simulink model "IEEE14Bus"  (R2024a)
settings: Solver=VariableStepAuto  StartTime=0.0  StopTime=10.0  RelTol=1e-3
values from neighbouring files (symbols this model uses):
  D1 = 2    [IEEE14Bus_params.m]
  M = 2*5.06    (= 10.12)    [IEEE14bus.m]    (also in IEEE14bus_revision.m; IEEE14bus_revision_new.m; IEEE14bus_revision_old.m; IEEE68withLocalSys14.m)
  Xd = 1.25    [IEEE14bus.m]    (also in IEEE14bus_revision.m; IEEE14bus_revision_new.m; IEEE14bus_revision_old.m; IEEE68withLocalSys14.m)
  Xq = 1.22    [IEEE14bus.m]    (also in IEEE14bus_revision.m; IEEE14bus_revision_new.m; IEEE14bus_revision_old.m; IEEE68withLocalSys14.m)
undefined symbols (not defined in the file or in its folder): ddTdo, ddTqo, ddXd, ddXq, Delta, dTdo, dXd, F, T1, T2, T3, T4, T5, T6, Xl
libraries: spsGroundLib x3, spsThreePhaseSeriesRLCBranchLib x3, spsThreePhaseParallelRLCLoadLib x2, spsLoadFlowBusLib x2, spsThreePhaseVIMeasurementLib x2, spsThreePhaseSourceLib x1, spsThreePhaseFaultLib x1, spsDC1AExcitationSystemLib x1, spsGenericPowerSystemStabilizerLib x1, spsST1AExcitationSystemLib x1, spsSynchronousMachinepuStandardLib x1, spsThreePhaseTransformerTwoWindingsLib x1
settings Model: Creator=byeonghwalee  LastModifiedBy=byeonghwalee

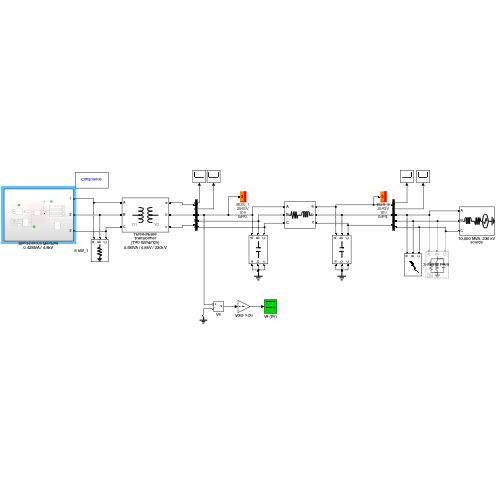
[thumbnail: Simulink's stored preview of the top-level diagram]
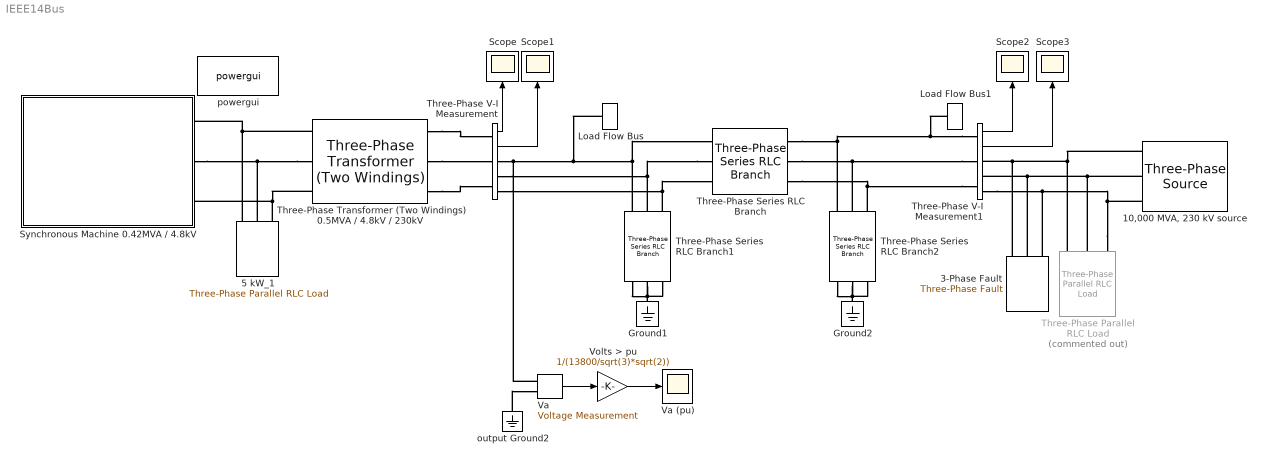
== system IEEE14Bus ==
  "10,000 MVA, 230 kV source" : spsThreePhaseSourceLib/Three-Phase Source  InternalConnection=Yg  VoltagePhases=off  Voltage=(230000)*1.00006  PhaseAngle=-0.77547  Voltage_phases=[25e3 25e3 25e3]/sqrt(3)  PhaseAngles_phases=[0 -120 +120]  Frequency=60  NonIdealSource=on  SpecifyImpedance=on  Resistance=0.529  Inductance=0.0140  ShortCircuitLevel=10000e6  BaseVoltage=230e3  XRratio=10  BusType=swing  Pref=0  Qref=0  Prefabc=[10e3, 10e3, 10e3]  Qrefabc=[0, 0, 0]  Qmin=-Inf  Qmax=Inf
  3-Phase Fault : spsThreePhaseFaultLib/Three-Phase Fault  InitialStates=0  FaultA=on  FaultB=on  FaultC=on  GroundFault=on  SwitchTimes=[3]  External=off  SwitchStatus=NaN  FaultResistance=1e-3  GroundResistance=1e-3  SnubberResistance=inf  SnubberCapacitance=inf  Measurements=None
  5 kW_1 : spsThreePhaseParallelRLCLoadLib/Three-Phase Parallel RLC Load  LConnTagsString=A|B|C  Configuration=Y (grounded)  NominalVoltage=230e3  Vabc=[1e3 1e3 1e3]  Vabcp=[1e3 1e3 1e3]  NominalFrequency=60  UnbalancedPower=off  ActivePower=100e3  InductivePower=0  CapacitivePower=0  Pabc=[10e3 9e3 11e3]  QLabc=[100 90 110]  QCabc=[100 90 110]  Pabcp=[10e3 9e3 11e3]  QLabcp=[100 90 110]  QCabcp=[100 90 110]  Measurements=None  LoadType=constant Z
  Ground1 : spsGroundLib/Ground  LConnTagsString=a
  Ground2 : spsGroundLib/Ground  LConnTagsString=a
  Load Flow Bus : spsLoadFlowBusLib/Load Flow Bus  LConnTagsString=a  Phases=single  Connectors=on one side  ID=BUS_1  Vbase=25e3  Vref=1  Vangle=0  VLF=1  VLFb=1  VLFc=1  angleLF=0  angleLFb=0  angleLFc=0
  Load Flow Bus1 : spsLoadFlowBusLib/Load Flow Bus  LConnTagsString=a  Phases=single  Connectors=on one side  ID=BUS_2  Vbase=25e3  Vref=1  Vangle=0  VLF=1  VLFb=1  VLFc=1  angleLF=0  angleLFb=0  angleLFc=0
  Scope{,1..3} (4 alike) : Scope
  Synchronous Machine 0.42MVA / 4.8kV : Subsystem
  Three-Phase Parallel RLC Load : spsThreePhaseParallelRLCLoadLib/Three-Phase Parallel RLC Load  Commented=on  LConnTagsString=A|B|C  Configuration=Y (grounded)  NominalVoltage=1000  Vabc=[1e3 1e3 1e3]  Vabcp=[1e3 1e3 1e3]  NominalFrequency=60  UnbalancedPower=off  ActivePower=10e3  InductivePower=100  CapacitivePower=100  Pabc=[10e3 9e3 11e3]  QLabc=[100 90 110]  QCabc=[100 90 110]  Pabcp=[10e3 9e3 11e3]  QLabcp=[100 90 110]  QCabcp=[100 90 110]  Measurements=None  LoadType=constant Z
  Three-Phase Series RLC Branch : spsThreePhaseSeriesRLCBranchLib/Three-Phase Series RLC Branch  LConnTagsString=A|B|C  RConnTagsString=A|B|C  BranchType=RL  Resistance=0.1375  Inductance=0.0698  Capacitance=1e-6  Measurements=None
  Three-Phase Series RLC Branch1 : spsThreePhaseSeriesRLCBranchLib/Three-Phase Series RLC Branch  LConnTagsString=A|B|C  RConnTagsString=A|B|C  BranchType=C  Resistance=1  Inductance=1e-3  Capacitance=(7.9377e-6)/2  Measurements=None
  Three-Phase Series RLC Branch2 : spsThreePhaseSeriesRLCBranchLib/Three-Phase Series RLC Branch  LConnTagsString=A|B|C  RConnTagsString=A|B|C  BranchType=C  Resistance=1  Inductance=1e-3  Capacitance=(7.9377e-6)/2  Measurements=None
  Three-Phase Transformer (Two Windings) 0.5MVA / 4.8kV / 230kV : spsThreePhaseTransformerTwoWindingsLib/Three-Phase Transformer (Two Windings)  Winding1Connection=Delta (D1)  Winding2Connection=Yg  CoreType=Three single-phase transformers  SetSaturation=off  Hysteresis=off  DataFile='hysteresis'  SetInitialFlux=off  Measurements=None  UNITS=pu  NominalPower=[ 0.5e6 , 60 ]  Winding1=[ 4.8e3 , 0.0027 , 0.08 ]  Winding2=[ 230e3 , 0.0027 , 0.08 ]  Rm=500  Lm=500  L0=0.5  Saturation=[ 0,0 ; 0.0024,1.2 ; 1.0,1.52 ]  InitialFluxes=[ 0.8 , -0.8 , 0.7 ]  BreakLoop=off  DiscreteSolver=Trapezoidal iterative  DataType=off  TransfoNumber=1
  Three-Phase V-I Measurement : spsThreePhaseVIMeasurementLib/Three-Phase V-I Measurement  VoltageMeasurement=phase-to-ground  SetLabelV=off  LabelV=Vabc  Vpu=off  VpuLL=off  CurrentMeasurement=yes  SetLabelI=off  LabelI=Iabc  Ipu=off  Pbase=100e6  Vbase=500e3  OutputType=Complex  PhasorSimulation=off  PSBequivalent=0
  Three-Phase V-I Measurement1 : spsThreePhaseVIMeasurementLib/Three-Phase V-I Measurement  VoltageMeasurement=phase-to-ground  SetLabelV=off  LabelV=Vabc  Vpu=off  VpuLL=off  CurrentMeasurement=yes  SetLabelI=off  LabelI=Iabc  Ipu=off  Pbase=100e6  Vbase=500e3  OutputType=Complex  PhasorSimulation=off  PSBequivalent=0
  Va : spsVoltageMeasurementLib/Voltage Measurement  Tag=PoWeRsYsTeMmEaSuReMeNt  PhasorSimulation=off  OutputType=Magnitude  PSBequivalent=0
  Va (pu) : Scope
  Volts > pu : Gain  Gain=1/(13800/sqrt(3)*sqrt(2))  SaturateOnIntegerOverflow=on  OutDataTypeStr=Inherit: Same as input  ParamDataTypeStr=Inherit: Same as input
  output Ground2 : spsGroundLib/Ground  LConnTagsString=a
  powergui : spspowerguiLib/powergui  Priority=1  SimulationMode=Continuous  SampleTime=0.001  frequency=60  Iterations=50  frequencyindice=60  Pbase=100e6  ErrMax=1e-4  UnitsV=kV  UnitsW=MW  buscounter=0  FunctionMessages=off  echomessages=off  EnableUseOfTLC=off  CurrentSourceSwitches=off  DisableSnubberDevices=off  DisableRonSwitches=off  DisableVfSwitches=off  DisplayEquations=off  AutomaticDiscreteSolvers=off  SolverType=Tustin/Backward Euler (TBE)  Interpol=off  ExternalGateDelay=off  methode=off  Ts=100  x0status=blocks  SPID=on  SwTol=0  HookPort=off  NonlinearTolerance=1e-4  nMaxIteration=100  ContinueOnMaxIteration=off  RestoreLinks=warning  ResistiveCurrentMeasurement=off  Frange=[0:2:500]  Ylog=off  Xlog=on  ShowGrid=off  save=off  variable=ZData  structure=0  ZoomFFT=off  StartTime=0.0  cycles=1  DisplayStyle=1  fundamental=60  FreqAxis=off  MaxFrequency=1000  frequencyindicesteady=1  RmsSteady=1  display=off
  wires:
  Three-Phase V-I Measurement/1 -> Scope/1
  Volts > pu/1 -> Va (pu)/1
  Three-Phase V-I Measurement1/2 -> Scope3/1
  Three-Phase V-I Measurement/2 -> Scope1/1
  Three-Phase V-I Measurement1/1 -> Scope2/1
  Va/1 -> Volts > pu/1
  connections:
  Three-Phase V-I Measurement1/LConn2 -- Three-Phase Series RLC Branch/RConn2 -- Three-Phase Series RLC Branch2/LConn2
  Three-Phase Series RLC Branch1/RConn2 -- Ground1/LConn1 -- Three-Phase Series RLC Branch1/RConn3 -- Three-Phase Series RLC Branch1/RConn1
  Three-Phase V-I Measurement/RConn1 -- Three-Phase Series RLC Branch/LConn1 -- Three-Phase Series RLC Branch1/LConn1 -- Load Flow Bus/LConn1 -- Va/LConn1
  Three-Phase V-I Measurement1/RConn1 -- 3-Phase Fault/LConn1 -- Three-Phase Parallel RLC Load/LConn1 -- "10,000 MVA, 230 kV source"/RConn1
  Three-Phase V-I Measurement1/LConn3 -- Three-Phase Series RLC Branch/RConn3 -- Three-Phase Series RLC Branch2/LConn3
  Three-Phase V-I Measurement1/RConn2 -- Three-Phase Parallel RLC Load/LConn2 -- "10,000 MVA, 230 kV source"/RConn2 -- 3-Phase Fault/LConn2
  Three-Phase V-I Measurement1/LConn1 -- Three-Phase Series RLC Branch/RConn1 -- Three-Phase Series RLC Branch2/LConn1 -- Load Flow Bus1/LConn1
  Three-Phase V-I Measurement/RConn3 -- Three-Phase Series RLC Branch1/LConn3 -- Three-Phase Series RLC Branch/LConn3
  Three-Phase Parallel RLC Load/LConn3 -- Three-Phase V-I Measurement1/RConn3 -- 3-Phase Fault/LConn3 -- "10,000 MVA, 230 kV source"/RConn3
  Three-Phase Series RLC Branch/LConn2 -- Three-Phase Series RLC Branch1/LConn2 -- Three-Phase V-I Measurement/RConn2
  Synchronous Machine 0.42MVA / 4.8kV/RConn3 -- Three-Phase Transformer (Two Windings) 0.5MVA / 4.8kV / 230kV/LConn3 -- 5 kW_1/LConn3
  Three-Phase Series RLC Branch2/RConn2 -- Ground2/LConn1 -- Three-Phase Series RLC Branch2/RConn1 -- Three-Phase Series RLC Branch2/RConn3
  Synchronous Machine 0.42MVA / 4.8kV/RConn1 -- Three-Phase Transformer (Two Windings) 0.5MVA / 4.8kV / 230kV/LConn1 -- 5 kW_1/LConn1
  Three-Phase Transformer (Two Windings) 0.5MVA / 4.8kV / 230kV/LConn2 -- Synchronous Machine 0.42MVA / 4.8kV/RConn2 -- 5 kW_1/LConn2
  Three-Phase Transformer (Two Windings) 0.5MVA / 4.8kV / 230kV/RConn1 -- Three-Phase V-I Measurement/LConn1
  Three-Phase Transformer (Two Windings) 0.5MVA / 4.8kV / 230kV/RConn2 -- Three-Phase V-I Measurement/LConn2
  Three-Phase Transformer (Two Windings) 0.5MVA / 4.8kV / 230kV/RConn3 -- Three-Phase V-I Measurement/LConn3
  output Ground2/LConn1 -- Va/LConn2

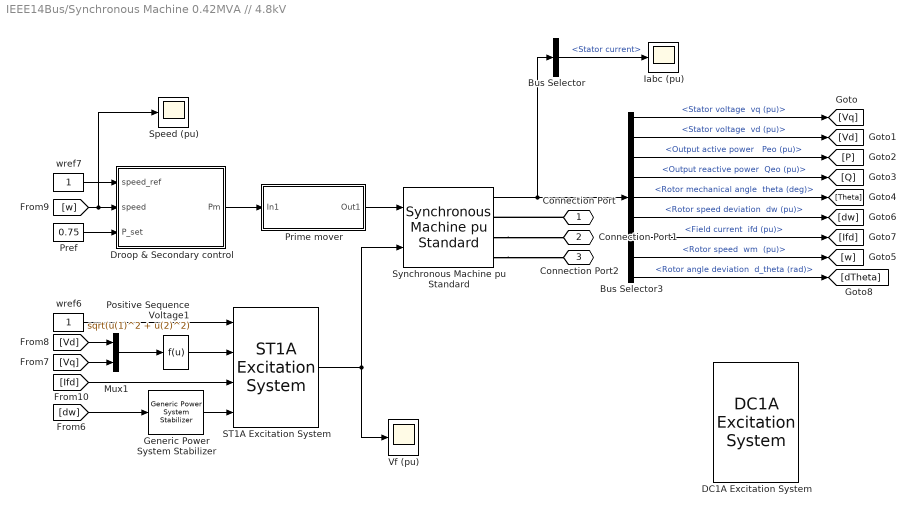
== system IEEE14Bus/Synchronous Machine 0.42MVA // 4.8kV ==
  " Iabc (pu)" : Scope
  " Speed (pu)" : Scope
  Bus Selector : BusSelector  OutputSignals=Stator current
  Bus Selector3 : BusSelector  OutputSignals="dq0 components.Stator voltage  vq (pu),dq0 components.Stator voltage  vd (pu),Output active power   Peo (pu),Output reactive power  Qeo (pu),Mechanical.Rotor mechanical angle  theta (deg),Mechanical.Rotor speed deviation  dw (pu),dq0 components.Field current  ifd (pu),Mechanical.Rotor speed  wm  (pu),Mechanical.Rotor angle deviation  d_theta (rad)"
  DC1A Excitation System : spsDC1AExcitationSystemLib/DC1A Excitation System  Tr=20e-3  KaTa=[46 0.06]  VRminmax=[-0.9 1.0]  KfTf=[0.05 1.5]  TbTc=[0 0]  KeTe=[0.05 0.46]  Efd12=[3.1 2.3]  SeEfd12=[0.33 0.10]  v0=[1 1]  TsBlock=0
      settings: LibrarySourceBlock=|
      | sps_lib/Electrical Machines/Synchronous Machine Control/DC1A
      | Excitation System
  Droop & Secondary control : Subsystem
  Generic Power System Stabilizer : spsGenericPowerSystemStabilizerLib/Generic Power System Stabilizer  Tsensor=30e-3  K=15  Twashout=1  Tleadlag1=[50e-3 20e-3]  Tleadlag2=[3 5.4]  VSlimits=[-0.15 0.15]  Vinit=0  Plot_On=off  MagdB_On=on  FreqRange=logspace(-2,2,500)
      settings: LibrarySourceBlock=|
      | sps_lib/Electrical Machines/Synchronous Machine Control/Generic
      | Power System Stabilizer
  Mux1 : Mux  Inputs=2
  Positive Sequence Voltage1 : Fcn  Expr=sqrt(u(1)^2 + u(2)^2)
  Pref : Constant  Value=0.75
  Prime mover : Subsystem
  ST1A Excitation System : spsST1AExcitationSystemLib/ST1A Excitation System  Tr=20e-3  KaTa=[210 0.001]  VIminmax=[-999 +999]  VAminmax=[-999 999]  VRminmax=[-6.0 6.43]  KfTf=[0.001 1]  TbTc=[0 0 0 0]  KLR=1  ILR=2  Kc=0.038  v0=[1 1]  TsBlock=0
      settings: LibrarySourceBlock=|
      | sps_lib/Electrical Machines/Synchronous Machine Control/ST1A
      | Excitation System
  Synchronous Machine pu Standard : spsSynchronousMachinepuStandardLib/Synchronous Machine pu Standard  PresetModel=No  MechanicalLoad=Mechanical power Pm  ShowDetailedParameters=on  RotorType=Salient-pole  Units=per unit standard parameters  MeasurementBus=off  NominalParameters=[0.42e6 4.8e3 60]  Reactances1=[ 1.81, 0.3, 0.23, 1.76, 0.65, 0.25, 0.15 ]  Reactances2=[Xd dXd ddXd Xq ddXq Xl]  dAxisTimeConstants=Open-circuit  qAxisTimeConstants=Open-circuit  TimeConstants1="[ dTdo ddTdo  ddTqo]"  TimeConstants2=[ 8.0, 0.03, 1.0, 0.07 ]  TimeConstants3="[  4.49  0.0681  0.0513  ]"  TimeConstants4=[ 8.0, 0.03, 0.3371, 0.0295 ]  TimeConstants5=[ 1.01, 0.053, 0.1 ]  TimeConstants6=[ 1.3201, 0.023, 1.0, 0.07 ]  TimeConstants7=[0.012 0.003 0.003]  TimeConstants8=[ 1.3201, 0.0231, 0.3371, 0.0295 ]  StatorResistance=Rs  Mechanical=[M F 2]  PolePairs=20  InitialConditions="[ 0  0  0  0  0  0  -120  120  1 ]"  SetSaturation=off  Saturation=[0.6404,0.7127,0.8441,0.9214,0.9956,1.082,1.19,1.316,1.457;0.7,0.7698,0.8872,0.9466,0.9969,1.046,1.1,1.151,1.201]  LoadFlowParameters=[1 0 0 0 0]  TsPowergui=0  TsBlock=-1  IterativeModel=Trapezoidal non iterative  IterativeDiscreteModel=Trapezoidal non iterative  BusType=PV  Pref=300e3  Qref=0  Qmin=-inf  Qmax=inf  PLF=0  QLF=0
  Vf (pu) : Scope
  wref6 : Constant
  wref7 : Constant
  Connection Port : PMIOPort  Side=Right
  Connection Port1 : PMIOPort  Port=2  Side=Right
  Connection Port2 : PMIOPort  Port=3  Side=Right
  wires:
  Bus Selector3/9 -> [dTheta]  "<Rotor angle deviation  d_theta (rad)>"
  Bus Selector3/8 -> [w]  "<Rotor speed  wm  (pu)>"
  Bus Selector3/1 -> [Vq]  "<Stator voltage  vq (pu)>"
  Bus Selector3/7 -> [Ifd]  "<Field current  ifd (pu)>"
  Bus Selector3/2 -> [Vd]  "<Stator voltage  vd (pu)>"
  Bus Selector3/4 -> [Q]  "<Output reactive power  Qeo (pu)>"
  Bus Selector3/3 -> [P]  "<Output active power   Peo (pu)>"
  Bus Selector3/5 -> [Theta]  "<Rotor mechanical angle  theta (deg)>"
  Bus Selector3/6 -> [dw]  "<Rotor speed deviation  dw (pu)>"
  [Vd] -> Mux1/1
  Mux1/1 -> Positive Sequence Voltage1/1
  [Vq] -> Mux1/2
  [Ifd] -> ST1A Excitation System/3
  Generic Power System Stabilizer/1 -> ST1A Excitation System/4
  Positive Sequence Voltage1/1 -> ST1A Excitation System/2
  [dw] -> Generic Power System Stabilizer/1
  wref6/1 -> ST1A Excitation System/1
  wref7/1 -> Droop & Secondary control/1(speed_ref)
  Pref/1 -> Droop & Secondary control/3(P_set)
  Droop & Secondary control/1(Pm) -> Prime mover/1(In1)
  Prime mover/1(Out1) -> Synchronous Machine pu Standard/1
  [w] -> " Speed (pu)"/1, Droop & Secondary control/2(speed)
  ST1A Excitation System/1 -> Vf (pu)/1, Synchronous Machine pu Standard/2
  Bus Selector/1 -> " Iabc (pu)"/1  "<Stator current>"
  Synchronous Machine pu Standard/1 -> Bus Selector/1, Bus Selector3/1
  connections:
  Connection Port/RConn1 -- Synchronous Machine pu Standard/RConn1
  Synchronous Machine pu Standard/RConn2 -- Connection Port1/RConn1
  Synchronous Machine pu Standard/RConn3 -- Connection Port2/RConn1

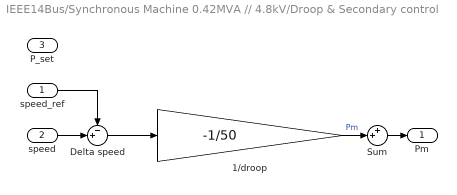
== system IEEE14Bus/Synchronous Machine 0.42MVA // 4.8kV/Droop & Secondary control ==
  speed_ref : Inport
  speed : Inport  Port=2
  P_set : Inport  Port=3
  1/droop : Gain  Gain=-1/50
  Delta speed : Sum  Inputs=-+|
  Sum : Sum  Inputs=++|
  Pm : Outport
  wires:
  speed_ref/1 -> Delta speed/1
  Delta speed/1 -> 1/droop/1
  speed/1 -> Delta speed/2
  1/droop/1 -> Sum/2  "Pm"
  Sum/1 -> Pm/1

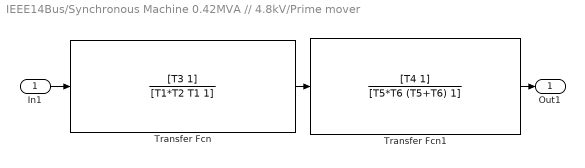
== system IEEE14Bus/Synchronous Machine 0.42MVA // 4.8kV/Prime mover ==
  In1 : Inport
  Transfer Fcn : TransferFcn  Numerator=[T3 1]  Denominator=[T1*T2 T1 1]
  Transfer Fcn1 : TransferFcn  Numerator=[T4 1]  Denominator=[T5*T6 (T5+T6) 1]
  Out1 : Outport
  wires:
  Transfer Fcn/1 -> Transfer Fcn1/1
  Transfer Fcn1/1 -> Out1/1
  In1/1 -> Transfer Fcn/1
